simulink model "ass"  (Simulink 6.5)
settings: Solver=ode45  StartTime=0.0  StopTime=10.0  RelTol=1e-3
libraries: cdsFilt x333, cdsPhase x144, cdsRfmIO x26, cdsOsc x18, cdsMuxMatrix x8, cdsEpicsOut x3, cdsEzCaRead x1, cdsEpicsIn x1, cdsBitwise x1, cdsParameters x1
(part 4 of 17)

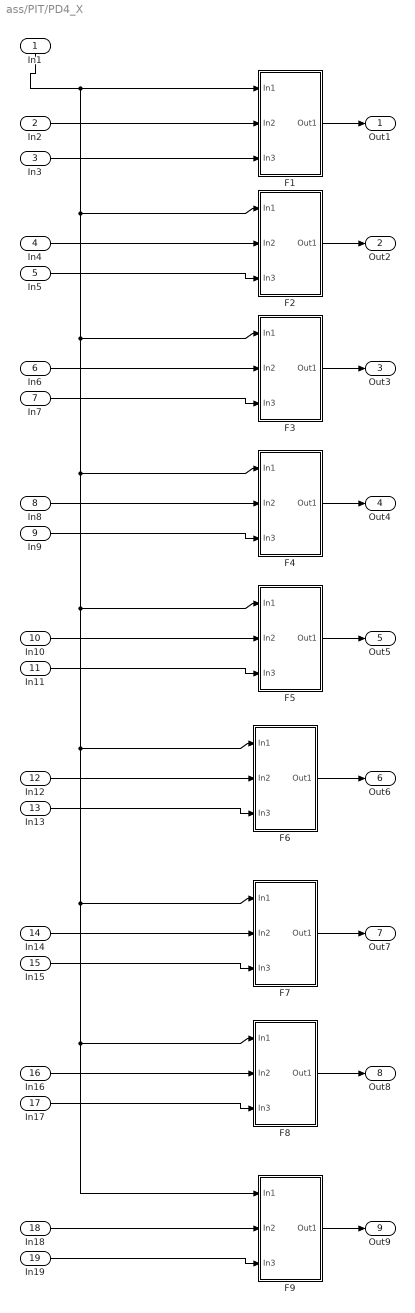
== system ass/PIT/PD4_X ==
  In1 : Inport  Orientation=down
  In2 : Inport  Port=2
  In3 : Inport  Port=3
  In4 : Inport  Port=4
  In5 : Inport  Port=5
  In6 : Inport  Port=6
  In7 : Inport  Port=7
  In8 : Inport  Port=8
  In9 : Inport  Port=9
  In10 : Inport  Port=10
  In11 : Inport  Port=11
  In12 : Inport  Port=12
  In13 : Inport  Port=13
  In14 : Inport  Port=14
  In15 : Inport  Port=15
  In16 : Inport  Port=16
  In17 : Inport  Port=17
  In18 : Inport  Port=18
  In19 : Inport  Port=19
  F1 : Subsystem
  F2 : Subsystem
  F3 : Subsystem
  F4 : Subsystem
  F5 : Subsystem
  F6 : Subsystem
  F7 : Subsystem
  F8 : Subsystem
  F9 : Subsystem
  Out1 : Outport
  Out2 : Outport  Port=2
  Out3 : Outport  Port=3
  Out4 : Outport  Port=4
  Out5 : Outport  Port=5
  Out6 : Outport  Port=6
  Out7 : Outport  Port=7
  Out8 : Outport  Port=8
  Out9 : Outport  Port=9
  wires:
  In1/1 -> F1/1(In1), F8/1(In1), F9/1(In1), F7/1(In1), F6/1(In1), F5/1(In1), F4/1(In1), F3/1(In1), F2/1(In1)
  In2/1 -> F1/2(In2)
  F1/1(Out1) -> Out1/1
  In3/1 -> F1/3(In3)
  In4/1 -> F2/2(In2)
  F2/1(Out1) -> Out2/1
  In5/1 -> F2/3(In3)
  In6/1 -> F3/2(In2)
  F3/1(Out1) -> Out3/1
  In7/1 -> F3/3(In3)
  In8/1 -> F4/2(In2)
  F4/1(Out1) -> Out4/1
  In9/1 -> F4/3(In3)
  In10/1 -> F5/2(In2)
  F5/1(Out1) -> Out5/1
  In11/1 -> F5/3(In3)
  In12/1 -> F6/2(In2)
  F6/1(Out1) -> Out6/1
  In13/1 -> F6/3(In3)
  In14/1 -> F7/2(In2)
  F7/1(Out1) -> Out7/1
  In15/1 -> F7/3(In3)
  In16/1 -> F8/2(In2)
  F8/1(Out1) -> Out8/1
  In17/1 -> F8/3(In3)
  In18/1 -> F9/2(In2)
  F9/1(Out1) -> Out9/1
  In19/1 -> F9/3(In3)

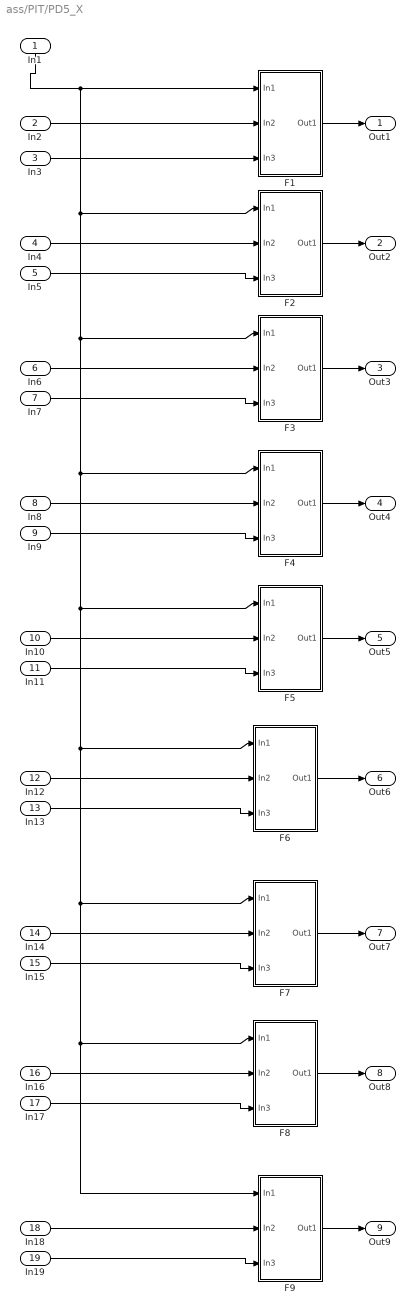
== system ass/PIT/PD5_X ==
  In1 : Inport  Orientation=down
  In2 : Inport  Port=2
  In3 : Inport  Port=3
  In4 : Inport  Port=4
  In5 : Inport  Port=5
  In6 : Inport  Port=6
  In7 : Inport  Port=7
  In8 : Inport  Port=8
  In9 : Inport  Port=9
  In10 : Inport  Port=10
  In11 : Inport  Port=11
  In12 : Inport  Port=12
  In13 : Inport  Port=13
  In14 : Inport  Port=14
  In15 : Inport  Port=15
  In16 : Inport  Port=16
  In17 : Inport  Port=17
  In18 : Inport  Port=18
  In19 : Inport  Port=19
  F1 : Subsystem
  F2 : Subsystem
  F3 : Subsystem
  F4 : Subsystem
  F5 : Subsystem
  F6 : Subsystem
  F7 : Subsystem
  F8 : Subsystem
  F9 : Subsystem
  Out1 : Outport
  Out2 : Outport  Port=2
  Out3 : Outport  Port=3
  Out4 : Outport  Port=4
  Out5 : Outport  Port=5
  Out6 : Outport  Port=6
  Out7 : Outport  Port=7
  Out8 : Outport  Port=8
  Out9 : Outport  Port=9
  wires:
  In1/1 -> F1/1(In1), F8/1(In1), F9/1(In1), F7/1(In1), F6/1(In1), F5/1(In1), F4/1(In1), F3/1(In1), F2/1(In1)
  In2/1 -> F1/2(In2)
  F1/1(Out1) -> Out1/1
  In3/1 -> F1/3(In3)
  In4/1 -> F2/2(In2)
  F2/1(Out1) -> Out2/1
  In5/1 -> F2/3(In3)
  In6/1 -> F3/2(In2)
  F3/1(Out1) -> Out3/1
  In7/1 -> F3/3(In3)
  In8/1 -> F4/2(In2)
  F4/1(Out1) -> Out4/1
  In9/1 -> F4/3(In3)
  In10/1 -> F5/2(In2)
  F5/1(Out1) -> Out5/1
  In11/1 -> F5/3(In3)
  In12/1 -> F6/2(In2)
  F6/1(Out1) -> Out6/1
  In13/1 -> F6/3(In3)
  In14/1 -> F7/2(In2)
  F7/1(Out1) -> Out7/1
  In15/1 -> F7/3(In3)
  In16/1 -> F8/2(In2)
  F8/1(Out1) -> Out8/1
  In17/1 -> F8/3(In3)
  In18/1 -> F9/2(In2)
  F9/1(Out1) -> Out9/1
  In19/1 -> F9/3(In3)

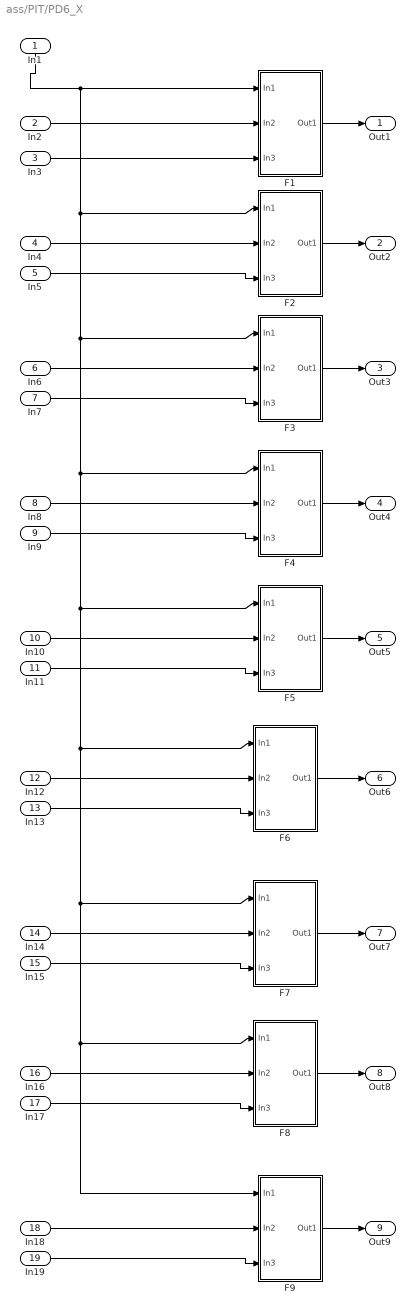
== system ass/PIT/PD6_X ==
  In1 : Inport  Orientation=down
  In2 : Inport  Port=2
  In3 : Inport  Port=3
  In4 : Inport  Port=4
  In5 : Inport  Port=5
  In6 : Inport  Port=6
  In7 : Inport  Port=7
  In8 : Inport  Port=8
  In9 : Inport  Port=9
  In10 : Inport  Port=10
  In11 : Inport  Port=11
  In12 : Inport  Port=12
  In13 : Inport  Port=13
  In14 : Inport  Port=14
  In15 : Inport  Port=15
  In16 : Inport  Port=16
  In17 : Inport  Port=17
  In18 : Inport  Port=18
  In19 : Inport  Port=19
  F1 : Subsystem
  F2 : Subsystem
  F3 : Subsystem
  F4 : Subsystem
  F5 : Subsystem
  F6 : Subsystem
  F7 : Subsystem
  F8 : Subsystem
  F9 : Subsystem
  Out1 : Outport
  Out2 : Outport  Port=2
  Out3 : Outport  Port=3
  Out4 : Outport  Port=4
  Out5 : Outport  Port=5
  Out6 : Outport  Port=6
  Out7 : Outport  Port=7
  Out8 : Outport  Port=8
  Out9 : Outport  Port=9
  wires:
  In1/1 -> F1/1(In1), F8/1(In1), F9/1(In1), F7/1(In1), F6/1(In1), F5/1(In1), F4/1(In1), F3/1(In1), F2/1(In1)
  In2/1 -> F1/2(In2)
  F1/1(Out1) -> Out1/1
  In3/1 -> F1/3(In3)
  In4/1 -> F2/2(In2)
  F2/1(Out1) -> Out2/1
  In5/1 -> F2/3(In3)
  In6/1 -> F3/2(In2)
  F3/1(Out1) -> Out3/1
  In7/1 -> F3/3(In3)
  In8/1 -> F4/2(In2)
  F4/1(Out1) -> Out4/1
  In9/1 -> F4/3(In3)
  In10/1 -> F5/2(In2)
  F5/1(Out1) -> Out5/1
  In11/1 -> F5/3(In3)
  In12/1 -> F6/2(In2)
  F6/1(Out1) -> Out6/1
  In13/1 -> F6/3(In3)
  In14/1 -> F7/2(In2)
  F7/1(Out1) -> Out7/1
  In15/1 -> F7/3(In3)
  In16/1 -> F8/2(In2)
  F8/1(Out1) -> Out8/1
  In17/1 -> F8/3(In3)
  In18/1 -> F9/2(In2)
  F9/1(Out1) -> Out9/1
  In19/1 -> F9/3(In3)

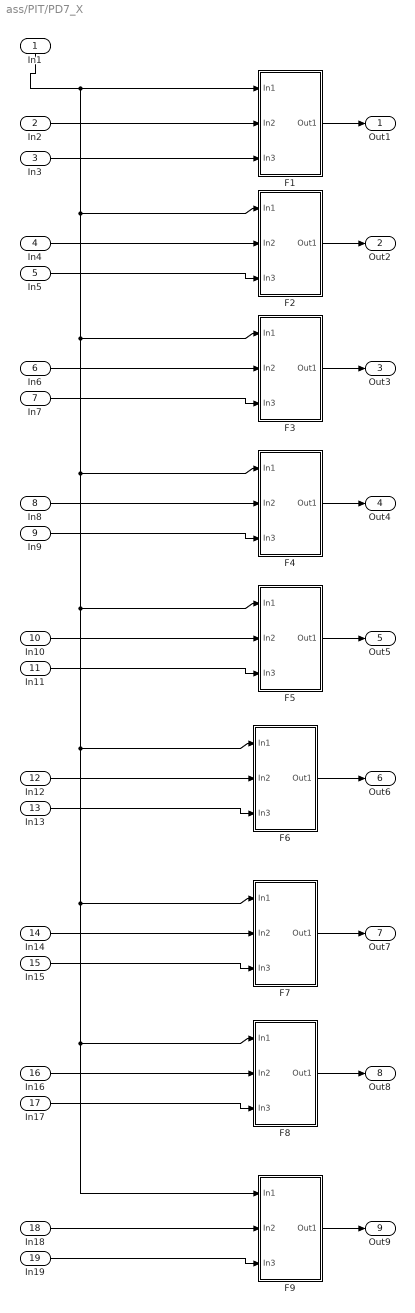
== system ass/PIT/PD7_X ==
  In1 : Inport  Orientation=down
  In2 : Inport  Port=2
  In3 : Inport  Port=3
  In4 : Inport  Port=4
  In5 : Inport  Port=5
  In6 : Inport  Port=6
  In7 : Inport  Port=7
  In8 : Inport  Port=8
  In9 : Inport  Port=9
  In10 : Inport  Port=10
  In11 : Inport  Port=11
  In12 : Inport  Port=12
  In13 : Inport  Port=13
  In14 : Inport  Port=14
  In15 : Inport  Port=15
  In16 : Inport  Port=16
  In17 : Inport  Port=17
  In18 : Inport  Port=18
  In19 : Inport  Port=19
  F1 : Subsystem
  F2 : Subsystem
  F3 : Subsystem
  F4 : Subsystem
  F5 : Subsystem
  F6 : Subsystem
  F7 : Subsystem
  F8 : Subsystem
  F9 : Subsystem
  Out1 : Outport
  Out2 : Outport  Port=2
  Out3 : Outport  Port=3
  Out4 : Outport  Port=4
  Out5 : Outport  Port=5
  Out6 : Outport  Port=6
  Out7 : Outport  Port=7
  Out8 : Outport  Port=8
  Out9 : Outport  Port=9
  wires:
  In1/1 -> F1/1(In1), F8/1(In1), F9/1(In1), F7/1(In1), F6/1(In1), F5/1(In1), F4/1(In1), F3/1(In1), F2/1(In1)
  In2/1 -> F1/2(In2)
  F1/1(Out1) -> Out1/1
  In3/1 -> F1/3(In3)
  In4/1 -> F2/2(In2)
  F2/1(Out1) -> Out2/1
  In5/1 -> F2/3(In3)
  In6/1 -> F3/2(In2)
  F3/1(Out1) -> Out3/1
  In7/1 -> F3/3(In3)
  In8/1 -> F4/2(In2)
  F4/1(Out1) -> Out4/1
  In9/1 -> F4/3(In3)
  In10/1 -> F5/2(In2)
  F5/1(Out1) -> Out5/1
  In11/1 -> F5/3(In3)
  In12/1 -> F6/2(In2)
  F6/1(Out1) -> Out6/1
  In13/1 -> F6/3(In3)
  In14/1 -> F7/2(In2)
  F7/1(Out1) -> Out7/1
  In15/1 -> F7/3(In3)
  In16/1 -> F8/2(In2)
  F8/1(Out1) -> Out8/1
  In17/1 -> F8/3(In3)
  In18/1 -> F9/2(In2)
  F9/1(Out1) -> Out9/1
  In19/1 -> F9/3(In3)

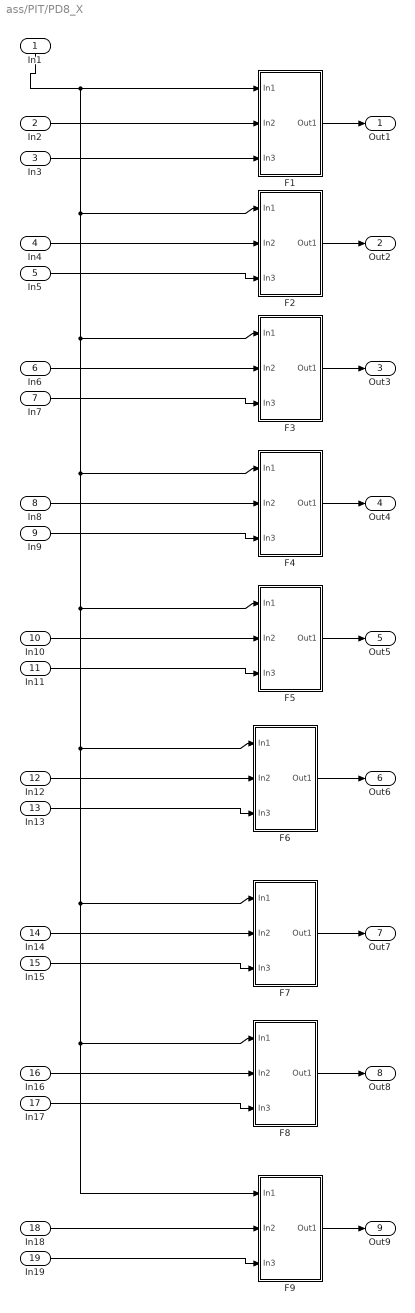
== system ass/PIT/PD8_X ==
  In1 : Inport  Orientation=down
  In2 : Inport  Port=2
  In3 : Inport  Port=3
  In4 : Inport  Port=4
  In5 : Inport  Port=5
  In6 : Inport  Port=6
  In7 : Inport  Port=7
  In8 : Inport  Port=8
  In9 : Inport  Port=9
  In10 : Inport  Port=10
  In11 : Inport  Port=11
  In12 : Inport  Port=12
  In13 : Inport  Port=13
  In14 : Inport  Port=14
  In15 : Inport  Port=15
  In16 : Inport  Port=16
  In17 : Inport  Port=17
  In18 : Inport  Port=18
  In19 : Inport  Port=19
  F1 : Subsystem
  F2 : Subsystem
  F3 : Subsystem
  F4 : Subsystem
  F5 : Subsystem
  F6 : Subsystem
  F7 : Subsystem
  F8 : Subsystem
  F9 : Subsystem
  Out1 : Outport
  Out2 : Outport  Port=2
  Out3 : Outport  Port=3
  Out4 : Outport  Port=4
  Out5 : Outport  Port=5
  Out6 : Outport  Port=6
  Out7 : Outport  Port=7
  Out8 : Outport  Port=8
  Out9 : Outport  Port=9
  wires:
  In1/1 -> F1/1(In1), F8/1(In1), F9/1(In1), F7/1(In1), F6/1(In1), F5/1(In1), F4/1(In1), F3/1(In1), F2/1(In1)
  In2/1 -> F1/2(In2)
  F1/1(Out1) -> Out1/1
  In3/1 -> F1/3(In3)
  In4/1 -> F2/2(In2)
  F2/1(Out1) -> Out2/1
  In5/1 -> F2/3(In3)
  In6/1 -> F3/2(In2)
  F3/1(Out1) -> Out3/1
  In7/1 -> F3/3(In3)
  In8/1 -> F4/2(In2)
  F4/1(Out1) -> Out4/1
  In9/1 -> F4/3(In3)
  In10/1 -> F5/2(In2)
  F5/1(Out1) -> Out5/1
  In11/1 -> F5/3(In3)
  In12/1 -> F6/2(In2)
  F6/1(Out1) -> Out6/1
  In13/1 -> F6/3(In3)
  In14/1 -> F7/2(In2)
  F7/1(Out1) -> Out7/1
  In15/1 -> F7/3(In3)
  In16/1 -> F8/2(In2)
  F8/1(Out1) -> Out8/1
  In17/1 -> F8/3(In3)
  In18/1 -> F9/2(In2)
  F9/1(Out1) -> Out9/1
  In19/1 -> F9/3(In3)

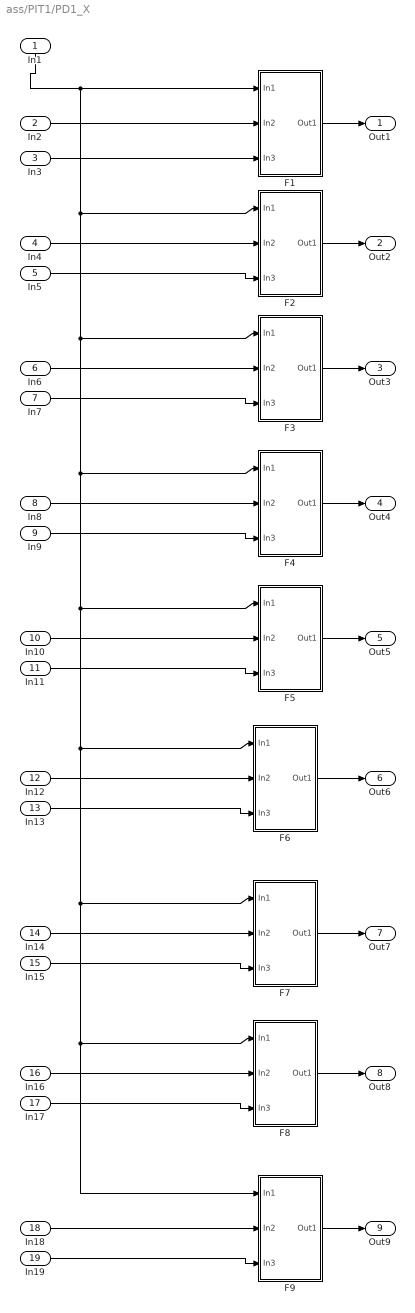
== system ass/PIT1/PD1_X ==
  In1 : Inport  Orientation=down
  In2 : Inport  Port=2
  In3 : Inport  Port=3
  In4 : Inport  Port=4
  In5 : Inport  Port=5
  In6 : Inport  Port=6
  In7 : Inport  Port=7
  In8 : Inport  Port=8
  In9 : Inport  Port=9
  In10 : Inport  Port=10
  In11 : Inport  Port=11
  In12 : Inport  Port=12
  In13 : Inport  Port=13
  In14 : Inport  Port=14
  In15 : Inport  Port=15
  In16 : Inport  Port=16
  In17 : Inport  Port=17
  In18 : Inport  Port=18
  In19 : Inport  Port=19
  F1 : Subsystem
  F2 : Subsystem
  F3 : Subsystem
  F4 : Subsystem
  F5 : Subsystem
  F6 : Subsystem
  F7 : Subsystem
  F8 : Subsystem
  F9 : Subsystem
  Out1 : Outport
  Out2 : Outport  Port=2
  Out3 : Outport  Port=3
  Out4 : Outport  Port=4
  Out5 : Outport  Port=5
  Out6 : Outport  Port=6
  Out7 : Outport  Port=7
  Out8 : Outport  Port=8
  Out9 : Outport  Port=9
  wires:
  In1/1 -> F1/1(In1), F8/1(In1), F9/1(In1), F7/1(In1), F6/1(In1), F5/1(In1), F4/1(In1), F3/1(In1), F2/1(In1)
  In2/1 -> F1/2(In2)
  F1/1(Out1) -> Out1/1
  In3/1 -> F1/3(In3)
  In4/1 -> F2/2(In2)
  F2/1(Out1) -> Out2/1
  In5/1 -> F2/3(In3)
  In6/1 -> F3/2(In2)
  F3/1(Out1) -> Out3/1
  In7/1 -> F3/3(In3)
  In8/1 -> F4/2(In2)
  F4/1(Out1) -> Out4/1
  In9/1 -> F4/3(In3)
  In10/1 -> F5/2(In2)
  F5/1(Out1) -> Out5/1
  In11/1 -> F5/3(In3)
  In12/1 -> F6/2(In2)
  F6/1(Out1) -> Out6/1
  In13/1 -> F6/3(In3)
  In14/1 -> F7/2(In2)
  F7/1(Out1) -> Out7/1
  In15/1 -> F7/3(In3)
  In16/1 -> F8/2(In2)
  F8/1(Out1) -> Out8/1
  In17/1 -> F8/3(In3)
  In18/1 -> F9/2(In2)
  F9/1(Out1) -> Out9/1
  In19/1 -> F9/3(In3)

== system ass/PIT1/PD2_X ==
  In1 : Inport  Orientation=down
  In2 : Inport  Port=2
  In3 : Inport  Port=3
  In4 : Inport  Port=4
  In5 : Inport  Port=5
  In6 : Inport  Port=6
  In7 : Inport  Port=7
  In8 : Inport  Port=8
  In9 : Inport  Port=9
  In10 : Inport  Port=10
  In11 : Inport  Port=11
  In12 : Inport  Port=12
  In13 : Inport  Port=13
  In14 : Inport  Port=14
  In15 : Inport  Port=15
  In16 : Inport  Port=16
  In17 : Inport  Port=17
  In18 : Inport  Port=18
  In19 : Inport  Port=19
  F1 : Subsystem
  F2 : Subsystem
  F3 : Subsystem
  F4 : Subsystem
  F5 : Subsystem
  F6 : Subsystem
  F7 : Subsystem
  F8 : Subsystem
  F9 : Subsystem
  Out1 : Outport
  Out2 : Outport  Port=2
  Out3 : Outport  Port=3
  Out4 : Outport  Port=4
  Out5 : Outport  Port=5
  Out6 : Outport  Port=6
  Out7 : Outport  Port=7
  Out8 : Outport  Port=8
  Out9 : Outport  Port=9
  wires:
  In1/1 -> F1/1(In1), F8/1(In1), F9/1(In1), F7/1(In1), F6/1(In1), F5/1(In1), F4/1(In1), F3/1(In1), F2/1(In1)
  In2/1 -> F1/2(In2)
  F1/1(Out1) -> Out1/1
  In3/1 -> F1/3(In3)
  In4/1 -> F2/2(In2)
  F2/1(Out1) -> Out2/1
  In5/1 -> F2/3(In3)
  In6/1 -> F3/2(In2)
  F3/1(Out1) -> Out3/1
  In7/1 -> F3/3(In3)
  In8/1 -> F4/2(In2)
  F4/1(Out1) -> Out4/1
  In9/1 -> F4/3(In3)
  In10/1 -> F5/2(In2)
  F5/1(Out1) -> Out5/1
  In11/1 -> F5/3(In3)
  In12/1 -> F6/2(In2)
  F6/1(Out1) -> Out6/1
  In13/1 -> F6/3(In3)
  In14/1 -> F7/2(In2)
  F7/1(Out1) -> Out7/1
  In15/1 -> F7/3(In3)
  In16/1 -> F8/2(In2)
  F8/1(Out1) -> Out8/1
  In17/1 -> F8/3(In3)
  In18/1 -> F9/2(In2)
  F9/1(Out1) -> Out9/1
  In19/1 -> F9/3(In3)

== system ass/PIT1/PD3_X ==
  In1 : Inport  Orientation=down
  In2 : Inport  Port=2
  In3 : Inport  Port=3
  In4 : Inport  Port=4
  In5 : Inport  Port=5
  In6 : Inport  Port=6
  In7 : Inport  Port=7
  In8 : Inport  Port=8
  In9 : Inport  Port=9
  In10 : Inport  Port=10
  In11 : Inport  Port=11
  In12 : Inport  Port=12
  In13 : Inport  Port=13
  In14 : Inport  Port=14
  In15 : Inport  Port=15
  In16 : Inport  Port=16
  In17 : Inport  Port=17
  In18 : Inport  Port=18
  In19 : Inport  Port=19
  F1 : Subsystem
  F2 : Subsystem
  F3 : Subsystem
  F4 : Subsystem
  F5 : Subsystem
  F6 : Subsystem
  F7 : Subsystem
  F8 : Subsystem
  F9 : Subsystem
  Out1 : Outport
  Out2 : Outport  Port=2
  Out3 : Outport  Port=3
  Out4 : Outport  Port=4
  Out5 : Outport  Port=5
  Out6 : Outport  Port=6
  Out7 : Outport  Port=7
  Out8 : Outport  Port=8
  Out9 : Outport  Port=9
  wires:
  In1/1 -> F1/1(In1), F8/1(In1), F9/1(In1), F7/1(In1), F6/1(In1), F5/1(In1), F4/1(In1), F3/1(In1), F2/1(In1)
  In2/1 -> F1/2(In2)
  F1/1(Out1) -> Out1/1
  In3/1 -> F1/3(In3)
  In4/1 -> F2/2(In2)
  F2/1(Out1) -> Out2/1
  In5/1 -> F2/3(In3)
  In6/1 -> F3/2(In2)
  F3/1(Out1) -> Out3/1
  In7/1 -> F3/3(In3)
  In8/1 -> F4/2(In2)
  F4/1(Out1) -> Out4/1
  In9/1 -> F4/3(In3)
  In10/1 -> F5/2(In2)
  F5/1(Out1) -> Out5/1
  In11/1 -> F5/3(In3)
  In12/1 -> F6/2(In2)
  F6/1(Out1) -> Out6/1
  In13/1 -> F6/3(In3)
  In14/1 -> F7/2(In2)
  F7/1(Out1) -> Out7/1
  In15/1 -> F7/3(In3)
  In16/1 -> F8/2(In2)
  F8/1(Out1) -> Out8/1
  In17/1 -> F8/3(In3)
  In18/1 -> F9/2(In2)
  F9/1(Out1) -> Out9/1
  In19/1 -> F9/3(In3)

== system ass/PIT1/PD4_X ==
  In1 : Inport  Orientation=down
  In2 : Inport  Port=2
  In3 : Inport  Port=3
  In4 : Inport  Port=4
  In5 : Inport  Port=5
  In6 : Inport  Port=6
  In7 : Inport  Port=7
  In8 : Inport  Port=8
  In9 : Inport  Port=9
  In10 : Inport  Port=10
  In11 : Inport  Port=11
  In12 : Inport  Port=12
  In13 : Inport  Port=13
  In14 : Inport  Port=14
  In15 : Inport  Port=15
  In16 : Inport  Port=16
  In17 : Inport  Port=17
  In18 : Inport  Port=18
  In19 : Inport  Port=19
  F1 : Subsystem
  F2 : Subsystem
  F3 : Subsystem
  F4 : Subsystem
  F5 : Subsystem
  F6 : Subsystem
  F7 : Subsystem
  F8 : Subsystem
  F9 : Subsystem
  Out1 : Outport
  Out2 : Outport  Port=2
  Out3 : Outport  Port=3
  Out4 : Outport  Port=4
  Out5 : Outport  Port=5
  Out6 : Outport  Port=6
  Out7 : Outport  Port=7
  Out8 : Outport  Port=8
  Out9 : Outport  Port=9
  wires:
  In1/1 -> F1/1(In1), F8/1(In1), F9/1(In1), F7/1(In1), F6/1(In1), F5/1(In1), F4/1(In1), F3/1(In1), F2/1(In1)
  In2/1 -> F1/2(In2)
  F1/1(Out1) -> Out1/1
  In3/1 -> F1/3(In3)
  In4/1 -> F2/2(In2)
  F2/1(Out1) -> Out2/1
  In5/1 -> F2/3(In3)
  In6/1 -> F3/2(In2)
  F3/1(Out1) -> Out3/1
  In7/1 -> F3/3(In3)
  In8/1 -> F4/2(In2)
  F4/1(Out1) -> Out4/1
  In9/1 -> F4/3(In3)
  In10/1 -> F5/2(In2)
  F5/1(Out1) -> Out5/1
  In11/1 -> F5/3(In3)
  In12/1 -> F6/2(In2)
  F6/1(Out1) -> Out6/1
  In13/1 -> F6/3(In3)
  In14/1 -> F7/2(In2)
  F7/1(Out1) -> Out7/1
  In15/1 -> F7/3(In3)
  In16/1 -> F8/2(In2)
  F8/1(Out1) -> Out8/1
  In17/1 -> F8/3(In3)
  In18/1 -> F9/2(In2)
  F9/1(Out1) -> Out9/1
  In19/1 -> F9/3(In3)

== system ass/PIT1/PD5_X ==
  In1 : Inport  Orientation=down
  In2 : Inport  Port=2
  In3 : Inport  Port=3
  In4 : Inport  Port=4
  In5 : Inport  Port=5
  In6 : Inport  Port=6
  In7 : Inport  Port=7
  In8 : Inport  Port=8
  In9 : Inport  Port=9
  In10 : Inport  Port=10
  In11 : Inport  Port=11
  In12 : Inport  Port=12
  In13 : Inport  Port=13
  In14 : Inport  Port=14
  In15 : Inport  Port=15
  In16 : Inport  Port=16
  In17 : Inport  Port=17
  In18 : Inport  Port=18
  In19 : Inport  Port=19
  F1 : Subsystem
  F2 : Subsystem
  F3 : Subsystem
  F4 : Subsystem
  F5 : Subsystem
  F6 : Subsystem
  F7 : Subsystem
  F8 : Subsystem
  F9 : Subsystem
  Out1 : Outport
  Out2 : Outport  Port=2
  Out3 : Outport  Port=3
  Out4 : Outport  Port=4
  Out5 : Outport  Port=5
  Out6 : Outport  Port=6
  Out7 : Outport  Port=7
  Out8 : Outport  Port=8
  Out9 : Outport  Port=9
  wires:
  In1/1 -> F1/1(In1), F8/1(In1), F9/1(In1), F7/1(In1), F6/1(In1), F5/1(In1), F4/1(In1), F3/1(In1), F2/1(In1)
  In2/1 -> F1/2(In2)
  F1/1(Out1) -> Out1/1
  In3/1 -> F1/3(In3)
  In4/1 -> F2/2(In2)
  F2/1(Out1) -> Out2/1
  In5/1 -> F2/3(In3)
  In6/1 -> F3/2(In2)
  F3/1(Out1) -> Out3/1
  In7/1 -> F3/3(In3)
  In8/1 -> F4/2(In2)
  F4/1(Out1) -> Out4/1
  In9/1 -> F4/3(In3)
  In10/1 -> F5/2(In2)
  F5/1(Out1) -> Out5/1
  In11/1 -> F5/3(In3)
  In12/1 -> F6/2(In2)
  F6/1(Out1) -> Out6/1
  In13/1 -> F6/3(In3)
  In14/1 -> F7/2(In2)
  F7/1(Out1) -> Out7/1
  In15/1 -> F7/3(In3)
  In16/1 -> F8/2(In2)
  F8/1(Out1) -> Out8/1
  In17/1 -> F8/3(In3)
  In18/1 -> F9/2(In2)
  F9/1(Out1) -> Out9/1
  In19/1 -> F9/3(In3)

== system ass/PIT1/PD6_X ==
  In1 : Inport  Orientation=down
  In2 : Inport  Port=2
  In3 : Inport  Port=3
  In4 : Inport  Port=4
  In5 : Inport  Port=5
  In6 : Inport  Port=6
  In7 : Inport  Port=7
  In8 : Inport  Port=8
  In9 : Inport  Port=9
  In10 : Inport  Port=10
  In11 : Inport  Port=11
  In12 : Inport  Port=12
  In13 : Inport  Port=13
  In14 : Inport  Port=14
  In15 : Inport  Port=15
  In16 : Inport  Port=16
  In17 : Inport  Port=17
  In18 : Inport  Port=18
  In19 : Inport  Port=19
  F1 : Subsystem
  F2 : Subsystem
  F3 : Subsystem
  F4 : Subsystem
  F5 : Subsystem
  F6 : Subsystem
  F7 : Subsystem
  F8 : Subsystem
  F9 : Subsystem
  Out1 : Outport
  Out2 : Outport  Port=2
  Out3 : Outport  Port=3
  Out4 : Outport  Port=4
  Out5 : Outport  Port=5
  Out6 : Outport  Port=6
  Out7 : Outport  Port=7
  Out8 : Outport  Port=8
  Out9 : Outport  Port=9
  wires:
  In1/1 -> F1/1(In1), F8/1(In1), F9/1(In1), F7/1(In1), F6/1(In1), F5/1(In1), F4/1(In1), F3/1(In1), F2/1(In1)
  In2/1 -> F1/2(In2)
  F1/1(Out1) -> Out1/1
  In3/1 -> F1/3(In3)
  In4/1 -> F2/2(In2)
  F2/1(Out1) -> Out2/1
  In5/1 -> F2/3(In3)
  In6/1 -> F3/2(In2)
  F3/1(Out1) -> Out3/1
  In7/1 -> F3/3(In3)
  In8/1 -> F4/2(In2)
  F4/1(Out1) -> Out4/1
  In9/1 -> F4/3(In3)
  In10/1 -> F5/2(In2)
  F5/1(Out1) -> Out5/1
  In11/1 -> F5/3(In3)
  In12/1 -> F6/2(In2)
  F6/1(Out1) -> Out6/1
  In13/1 -> F6/3(In3)
  In14/1 -> F7/2(In2)
  F7/1(Out1) -> Out7/1
  In15/1 -> F7/3(In3)
  In16/1 -> F8/2(In2)
  F8/1(Out1) -> Out8/1
  In17/1 -> F8/3(In3)
  In18/1 -> F9/2(In2)
  F9/1(Out1) -> Out9/1
  In19/1 -> F9/3(In3)

== system ass/PIT1/PD7_X ==
  In1 : Inport  Orientation=down
  In2 : Inport  Port=2
  In3 : Inport  Port=3
  In4 : Inport  Port=4
  In5 : Inport  Port=5
  In6 : Inport  Port=6
  In7 : Inport  Port=7
  In8 : Inport  Port=8
  In9 : Inport  Port=9
  In10 : Inport  Port=10
  In11 : Inport  Port=11
  In12 : Inport  Port=12
  In13 : Inport  Port=13
  In14 : Inport  Port=14
  In15 : Inport  Port=15
  In16 : Inport  Port=16
  In17 : Inport  Port=17
  In18 : Inport  Port=18
  In19 : Inport  Port=19
  F1 : Subsystem
  F2 : Subsystem
  F3 : Subsystem
  F4 : Subsystem
  F5 : Subsystem
  F6 : Subsystem
  F7 : Subsystem
  F8 : Subsystem
  F9 : Subsystem
  Out1 : Outport
  Out2 : Outport  Port=2
  Out3 : Outport  Port=3
  Out4 : Outport  Port=4
  Out5 : Outport  Port=5
  Out6 : Outport  Port=6
  Out7 : Outport  Port=7
  Out8 : Outport  Port=8
  Out9 : Outport  Port=9
  wires:
  In1/1 -> F1/1(In1), F8/1(In1), F9/1(In1), F7/1(In1), F6/1(In1), F5/1(In1), F4/1(In1), F3/1(In1), F2/1(In1)
  In2/1 -> F1/2(In2)
  F1/1(Out1) -> Out1/1
  In3/1 -> F1/3(In3)
  In4/1 -> F2/2(In2)
  F2/1(Out1) -> Out2/1
  In5/1 -> F2/3(In3)
  In6/1 -> F3/2(In2)
  F3/1(Out1) -> Out3/1
  In7/1 -> F3/3(In3)
  In8/1 -> F4/2(In2)
  F4/1(Out1) -> Out4/1
  In9/1 -> F4/3(In3)
  In10/1 -> F5/2(In2)
  F5/1(Out1) -> Out5/1
  In11/1 -> F5/3(In3)
  In12/1 -> F6/2(In2)
  F6/1(Out1) -> Out6/1
  In13/1 -> F6/3(In3)
  In14/1 -> F7/2(In2)
  F7/1(Out1) -> Out7/1
  In15/1 -> F7/3(In3)
  In16/1 -> F8/2(In2)
  F8/1(Out1) -> Out8/1
  In17/1 -> F8/3(In3)
  In18/1 -> F9/2(In2)
  F9/1(Out1) -> Out9/1
  In19/1 -> F9/3(In3)

== system ass/PIT1/PD8_X ==
  In1 : Inport  Orientation=down
  In2 : Inport  Port=2
  In3 : Inport  Port=3
  In4 : Inport  Port=4
  In5 : Inport  Port=5
  In6 : Inport  Port=6
  In7 : Inport  Port=7
  In8 : Inport  Port=8
  In9 : Inport  Port=9
  In10 : Inport  Port=10
  In11 : Inport  Port=11
  In12 : Inport  Port=12
  In13 : Inport  Port=13
  In14 : Inport  Port=14
  In15 : Inport  Port=15
  In16 : Inport  Port=16
  In17 : Inport  Port=17
  In18 : Inport  Port=18
  In19 : Inport  Port=19
  F1 : Subsystem
  F2 : Subsystem
  F3 : Subsystem
  F4 : Subsystem
  F5 : Subsystem
  F6 : Subsystem
  F7 : Subsystem
  F8 : Subsystem
  F9 : Subsystem
  Out1 : Outport
  Out2 : Outport  Port=2
  Out3 : Outport  Port=3
  Out4 : Outport  Port=4
  Out5 : Outport  Port=5
  Out6 : Outport  Port=6
  Out7 : Outport  Port=7
  Out8 : Outport  Port=8
  Out9 : Outport  Port=9
  wires:
  In1/1 -> F1/1(In1), F8/1(In1), F9/1(In1), F7/1(In1), F6/1(In1), F5/1(In1), F4/1(In1), F3/1(In1), F2/1(In1)
  In2/1 -> F1/2(In2)
  F1/1(Out1) -> Out1/1
  In3/1 -> F1/3(In3)
  In4/1 -> F2/2(In2)
  F2/1(Out1) -> Out2/1
  In5/1 -> F2/3(In3)
  In6/1 -> F3/2(In2)
  F3/1(Out1) -> Out3/1
  In7/1 -> F3/3(In3)
  In8/1 -> F4/2(In2)
  F4/1(Out1) -> Out4/1
  In9/1 -> F4/3(In3)
  In10/1 -> F5/2(In2)
  F5/1(Out1) -> Out5/1
  In11/1 -> F5/3(In3)
  In12/1 -> F6/2(In2)
  F6/1(Out1) -> Out6/1
  In13/1 -> F6/3(In3)
  In14/1 -> F7/2(In2)
  F7/1(Out1) -> Out7/1
  In15/1 -> F7/3(In3)
  In16/1 -> F8/2(In2)
  F8/1(Out1) -> Out8/1
  In17/1 -> F8/3(In3)
  In18/1 -> F9/2(In2)
  F9/1(Out1) -> Out9/1
  In19/1 -> F9/3(In3)

== system ass/PIT/PD1_X/F1 ==
  In1 : Inport
  In2 : Inport  Port=2
  In3 : Inport  Port=3
  I : cdsFilt/Subsystem  Tag=cdsFilt  Description=|  SystemSampleTime=-1
      | Purpose:                                                                                                                                                                                                                                  
      | Standard CDS IIR filter module.                                                                                                                                                                                                           
      |                                                                                                                                                                                                                                           
      | Operation:                                                                                                                                                                                                                                
      | Consists of 10 second order section IIR filters, plus a ramped gain stage. In FE code, also provides pre-defined test points and excitation channel inputs. The filter coefficients are defined in the LIGO system using the 'foton' tool.
      |                                                                                                                                                                                                                                           
      | Usage:                                                                                                                                                                                                                                    
      | Name the part with the desired filter module name.
      settings: AttributesFormatString=%<Tag>
  PHASE : cdsPhase/Subsystem  Tag=cdsPhase  Description=Phase Rotator  SystemSampleTime=-1
      settings: AttributesFormatString=%<Tag>
  Product : Product  RndMeth=Zero
  Product1 : Product  RndMeth=Zero
  Q : cdsFilt/Subsystem  Tag=cdsFilt  Description=|  SystemSampleTime=-1
      | Purpose:                                                                                                                                                                                                                                  
      | Standard CDS IIR filter module.                                                                                                                                                                                                           
      |                                                                                                                                                                                                                                           
      | Operation:                                                                                                                                                                                                                                
      | Consists of 10 second order section IIR filters, plus a ramped gain stage. In FE code, also provides pre-defined test points and excitation channel inputs. The filter coefficients are defined in the LIGO system using the 'foton' tool.
      |                                                                                                                                                                                                                                           
      | Usage:                                                                                                                                                                                                                                    
      | Name the part with the desired filter module name.
      settings: AttributesFormatString=%<Tag>
  Terminator4 : Terminator
  Out1 : Outport
  wires:
  I/1 -> Out1/1
  PHASE/2 -> Q/1
  In1/1 -> Product/1, Product1/1
  In2/1 -> Product/2
  In3/1 -> Product1/2
  PHASE/1 -> I/1
  Product/1 -> PHASE/1
  Q/1 -> Terminator4/1
  Product1/1 -> PHASE/2

== system ass/PIT/PD1_X/F2 ==
  In1 : Inport
  In2 : Inport  Port=2
  In3 : Inport  Port=3
  I : cdsFilt/Subsystem  Tag=cdsFilt  Description=|  SystemSampleTime=-1
      | Purpose:                                                                                                                                                                                                                                  
      | Standard CDS IIR filter module.                                                                                                                                                                                                           
      |                                                                                                                                                                                                                                           
      | Operation:                                                                                                                                                                                                                                
      | Consists of 10 second order section IIR filters, plus a ramped gain stage. In FE code, also provides pre-defined test points and excitation channel inputs. The filter coefficients are defined in the LIGO system using the 'foton' tool.
      |                                                                                                                                                                                                                                           
      | Usage:                                                                                                                                                                                                                                    
      | Name the part with the desired filter module name.
      settings: AttributesFormatString=%<Tag>
  PHASE : cdsPhase/Subsystem  Tag=cdsPhase  Description=Phase Rotator  SystemSampleTime=-1
      settings: AttributesFormatString=%<Tag>
  Product : Product  RndMeth=Zero
  Product1 : Product  RndMeth=Zero
  Q : cdsFilt/Subsystem  Tag=cdsFilt  Description=|  SystemSampleTime=-1
      | Purpose:                                                                                                                                                                                                                                  
      | Standard CDS IIR filter module.                                                                                                                                                                                                           
      |                                                                                                                                                                                                                                           
      | Operation:                                                                                                                                                                                                                                
      | Consists of 10 second order section IIR filters, plus a ramped gain stage. In FE code, also provides pre-defined test points and excitation channel inputs. The filter coefficients are defined in the LIGO system using the 'foton' tool.
      |                                                                                                                                                                                                                                           
      | Usage:                                                                                                                                                                                                                                    
      | Name the part with the desired filter module name.
      settings: AttributesFormatString=%<Tag>
  Terminator4 : Terminator
  Out1 : Outport
  wires:
  I/1 -> Out1/1
  PHASE/2 -> Q/1
  In1/1 -> Product/1, Product1/1
  In2/1 -> Product/2
  In3/1 -> Product1/2
  PHASE/1 -> I/1
  Product/1 -> PHASE/1
  Q/1 -> Terminator4/1
  Product1/1 -> PHASE/2

== system ass/PIT/PD1_X/F3 ==
  In1 : Inport
  In2 : Inport  Port=2
  In3 : Inport  Port=3
  I : cdsFilt/Subsystem  Tag=cdsFilt  Description=|  SystemSampleTime=-1
      | Purpose:                                                                                                                                                                                                                                  
      | Standard CDS IIR filter module.                                                                                                                                                                                                           
      |                                                                                                                                                                                                                                           
      | Operation:                                                                                                                                                                                                                                
      | Consists of 10 second order section IIR filters, plus a ramped gain stage. In FE code, also provides pre-defined test points and excitation channel inputs. The filter coefficients are defined in the LIGO system using the 'foton' tool.
      |                                                                                                                                                                                                                                           
      | Usage:                                                                                                                                                                                                                                    
      | Name the part with the desired filter module name.
      settings: AttributesFormatString=%<Tag>
  PHASE : cdsPhase/Subsystem  Tag=cdsPhase  Description=Phase Rotator  SystemSampleTime=-1
      settings: AttributesFormatString=%<Tag>
  Product : Product  RndMeth=Zero
  Product1 : Product  RndMeth=Zero
  Q : cdsFilt/Subsystem  Tag=cdsFilt  Description=|  SystemSampleTime=-1
      | Purpose:                                                                                                                                                                                                                                  
      | Standard CDS IIR filter module.                                                                                                                                                                                                           
      |                                                                                                                                                                                                                                           
      | Operation:                                                                                                                                                                                                                                
      | Consists of 10 second order section IIR filters, plus a ramped gain stage. In FE code, also provides pre-defined test points and excitation channel inputs. The filter coefficients are defined in the LIGO system using the 'foton' tool.
      |                                                                                                                                                                                                                                           
      | Usage:                                                                                                                                                                                                                                    
      | Name the part with the desired filter module name.
      settings: AttributesFormatString=%<Tag>
  Terminator4 : Terminator
  Out1 : Outport
  wires:
  I/1 -> Out1/1
  PHASE/2 -> Q/1
  In1/1 -> Product/1, Product1/1
  In2/1 -> Product/2
  In3/1 -> Product1/2
  PHASE/1 -> I/1
  Product/1 -> PHASE/1
  Q/1 -> Terminator4/1
  Product1/1 -> PHASE/2

== system ass/PIT/PD1_X/F4 ==
  In1 : Inport
  In2 : Inport  Port=2
  In3 : Inport  Port=3
  I : cdsFilt/Subsystem  Tag=cdsFilt  Description=|  SystemSampleTime=-1
      | Purpose:                                                                                                                                                                                                                                  
      | Standard CDS IIR filter module.                                                                                                                                                                                                           
      |                                                                                                                                                                                                                                           
      | Operation:                                                                                                                                                                                                                                
      | Consists of 10 second order section IIR filters, plus a ramped gain stage. In FE code, also provides pre-defined test points and excitation channel inputs. The filter coefficients are defined in the LIGO system using the 'foton' tool.
      |                                                                                                                                                                                                                                           
      | Usage:                                                                                                                                                                                                                                    
      | Name the part with the desired filter module name.
      settings: AttributesFormatString=%<Tag>
  PHASE : cdsPhase/Subsystem  Tag=cdsPhase  Description=Phase Rotator  SystemSampleTime=-1
      settings: AttributesFormatString=%<Tag>
  Product : Product  RndMeth=Zero
  Product1 : Product  RndMeth=Zero
  Q : cdsFilt/Subsystem  Tag=cdsFilt  Description=|  SystemSampleTime=-1
      | Purpose:                                                                                                                                                                                                                                  
      | Standard CDS IIR filter module.                                                                                                                                                                                                           
      |                                                                                                                                                                                                                                           
      | Operation:                                                                                                                                                                                                                                
      | Consists of 10 second order section IIR filters, plus a ramped gain stage. In FE code, also provides pre-defined test points and excitation channel inputs. The filter coefficients are defined in the LIGO system using the 'foton' tool.
      |                                                                                                                                                                                                                                           
      | Usage:                                                                                                                                                                                                                                    
      | Name the part with the desired filter module name.
      settings: AttributesFormatString=%<Tag>
  Terminator4 : Terminator
  Out1 : Outport
  wires:
  I/1 -> Out1/1
  PHASE/2 -> Q/1
  In1/1 -> Product/1, Product1/1
  In2/1 -> Product/2
  In3/1 -> Product1/2
  PHASE/1 -> I/1
  Product/1 -> PHASE/1
  Q/1 -> Terminator4/1
  Product1/1 -> PHASE/2

== system ass/PIT/PD1_X/F5 ==
  In1 : Inport
  In2 : Inport  Port=2
  In3 : Inport  Port=3
  I : cdsFilt/Subsystem  Tag=cdsFilt  Description=|  SystemSampleTime=-1
      | Purpose:                                                                                                                                                                                                                                  
      | Standard CDS IIR filter module.                                                                                                                                                                                                           
      |                                                                                                                                                                                                                                           
      | Operation:                                                                                                                                                                                                                                
      | Consists of 10 second order section IIR filters, plus a ramped gain stage. In FE code, also provides pre-defined test points and excitation channel inputs. The filter coefficients are defined in the LIGO system using the 'foton' tool.
      |                                                                                                                                                                                                                                           
      | Usage:                                                                                                                                                                                                                                    
      | Name the part with the desired filter module name.
      settings: AttributesFormatString=%<Tag>
  PHASE : cdsPhase/Subsystem  Tag=cdsPhase  Description=Phase Rotator  SystemSampleTime=-1
      settings: AttributesFormatString=%<Tag>
  Product : Product  RndMeth=Zero
  Product1 : Product  RndMeth=Zero
  Q : cdsFilt/Subsystem  Tag=cdsFilt  Description=|  SystemSampleTime=-1
      | Purpose:                                                                                                                                                                                                                                  
      | Standard CDS IIR filter module.                                                                                                                                                                                                           
      |                                                                                                                                                                                                                                           
      | Operation:                                                                                                                                                                                                                                
      | Consists of 10 second order section IIR filters, plus a ramped gain stage. In FE code, also provides pre-defined test points and excitation channel inputs. The filter coefficients are defined in the LIGO system using the 'foton' tool.
      |                                                                                                                                                                                                                                           
      | Usage:                                                                                                                                                                                                                                    
      | Name the part with the desired filter module name.
      settings: AttributesFormatString=%<Tag>
  Terminator4 : Terminator
  Out1 : Outport
  wires:
  I/1 -> Out1/1
  PHASE/2 -> Q/1
  In1/1 -> Product/1, Product1/1
  In2/1 -> Product/2
  In3/1 -> Product1/2
  PHASE/1 -> I/1
  Product/1 -> PHASE/1
  Q/1 -> Terminator4/1
  Product1/1 -> PHASE/2

== system ass/PIT/PD1_X/F6 ==
  In1 : Inport
  In2 : Inport  Port=2
  In3 : Inport  Port=3
  I : cdsFilt/Subsystem  Tag=cdsFilt  Description=|  SystemSampleTime=-1
      | Purpose:                                                                                                                                                                                                                                  
      | Standard CDS IIR filter module.                                                                                                                                                                                                           
      |                                                                                                                                                                                                                                           
      | Operation:                                                                                                                                                                                                                                
      | Consists of 10 second order section IIR filters, plus a ramped gain stage. In FE code, also provides pre-defined test points and excitation channel inputs. The filter coefficients are defined in the LIGO system using the 'foton' tool.
      |                                                                                                                                                                                                                                           
      | Usage:                                                                                                                                                                                                                                    
      | Name the part with the desired filter module name.
      settings: AttributesFormatString=%<Tag>
  PHASE : cdsPhase/Subsystem  Tag=cdsPhase  Description=Phase Rotator  SystemSampleTime=-1
      settings: AttributesFormatString=%<Tag>
  Product : Product  RndMeth=Zero
  Product1 : Product  RndMeth=Zero
  Q : cdsFilt/Subsystem  Tag=cdsFilt  Description=|  SystemSampleTime=-1
      | Purpose:                                                                                                                                                                                                                                  
      | Standard CDS IIR filter module.                                                                                                                                                                                                           
      |                                                                                                                                                                                                                                           
      | Operation:                                                                                                                                                                                                                                
      | Consists of 10 second order section IIR filters, plus a ramped gain stage. In FE code, also provides pre-defined test points and excitation channel inputs. The filter coefficients are defined in the LIGO system using the 'foton' tool.
      |                                                                                                                                                                                                                                           
      | Usage:                                                                                                                                                                                                                                    
      | Name the part with the desired filter module name.
      settings: AttributesFormatString=%<Tag>
  Terminator4 : Terminator
  Out1 : Outport
  wires:
  I/1 -> Out1/1
  PHASE/2 -> Q/1
  In1/1 -> Product/1, Product1/1
  In2/1 -> Product/2
  In3/1 -> Product1/2
  PHASE/1 -> I/1
  Product/1 -> PHASE/1
  Q/1 -> Terminator4/1
  Product1/1 -> PHASE/2
